simulink model "PassCarModel_RL_config"  (R2024b)
settings: Solver=FixedStepAuto  StartTime=0.0  StopTime=Tf  FixedStep=.001  RelTol=1e-2
StartFcn:
  | %tic
StopFcn:
  | %toc
model workspace (MAT data in the model file):
  AverageTimeInterval = 0.5
  Downshift_Speeds = [9.5625 12.9375 16.3125 19.6875 23.0625 26.4375 29.8125 33.1875 36.5625 39.9375 43.3125 46.6875 ... (28 elements, 4x7)]
  EEC_Counter : Simulink.Parameter (value not decoded)
  EngRevLim = 7000
  FuzzOffset : Simulink.Parameter (value not decoded)
  FuzzRange : Simulink.Parameter (value not decoded)
  Fuzzing : Simulink.Parameter (value not decoded)
  Pedal_Positions = [0.1 0.4 0.5 0.9]
  TrackPoints = [0 36.336 72.672 109.008 145.344 181.68 218.016 254.352 290.688 327.024 363.36 403.196036522 ... (360 elements, 120x3)]
  Upshift_Speeds = [12.9375 16.3125 19.6875 33 26.4375 29.8125 33.1875 52.5 39.9375 43.3125 46.6875 77.25 ... (28 elements, 4x7)]
  VEH : object (value not decoded)
  gradbp : Simulink.Parameter (value not decoded)
  origin : Simulink.Parameter (value not decoded)
  rayDirections = [0 0 0 0 0 0 0 0 0 0 0 0 ... (363 elements, 121x3)]
  rayLengths = [20 20 20 20 20 20 20 20 20 20 20 20 ... (121 elements, 121x1)]
  rayOrigins = [0.5 0.4 0.3 0.2 0.1 0 -0.1 -0.2 -0.3 -0.4 -0.5 0.5 ... (363 elements, 121x3)]
  theta : Simulink.Parameter (value not decoded)
  totalDistance : Simulink.Parameter (value not decoded)
  vel_profile3 : Simulink.Parameter (value not decoded)
  xEast : Simulink.Parameter (value not decoded)
  yNorth : Simulink.Parameter (value not decoded)
symbols that are objects in the model workspace (value not decoded): gradbp, origin, theta, totalDistance, VEH, vel_profile3, xEast, yNorth
undefined symbols (not defined in the file or in its folder): DecelR, DiscIntNeverNeededParam, dspblkCoreblockFVToolHelper, FO_max, FO_min, FR_max, FR_min, gcbh, ODevR, Sim3dSensor, Ts
libraries: simulink x20, dspstat3 x8, autolibutils x6, sim3dgroundtruthsensorlib x2, rllib x1, slpidlib x1, autolibtranscontrolscommon x1, vehdynlibdriver x1, sharedtransform x1, vehdynlibviscommon x1, vehdynlibsens x1
(part 2 of 5)

== system PassCarModel_RL_config/Controllers and CAN network/CAN/BrakeController ==
  Fuzzing : Inport
  VehDataBus : Inport  Port=2
  Bus Creator1 : BusCreator  Inputs=6
  Bus Selector3 : BusSelector  OutputSignals=Cntrl.Brake.ABSFlag,Cntrl.Brake.TCSFlag,Driveline.BrkPrs,Cntrl.Brake.BrkPrsCmd,Wheels.TireFrame.Omega
  EBC1 : Subsystem
  EBC2 : Subsystem
  EBC3 : Subsystem
  EBC4 : Subsystem
  NoiseGenerator : Subsystem
  BrakeController : Outport
  wires:
  VehDataBus/1 -> NoiseGenerator/1(In1), Bus Selector3/1
  Bus Selector3/1 -> EBC1/1(ABSFlagIn)  "<ABSFlag>"
  Bus Selector3/2 -> EBC1/2(TCSFlagIn)  "<TCSFlag>"
  EBC1/1(ABSFlag) -> Bus Creator1/1
  Bus Selector3/3 -> EBC2/1(<BrkPrs>)  "<BrkPrs>"
  EBC2/1(BrkPrs) -> Bus Creator1/3
  Bus Selector3/4 -> EBC3/1(<BrkPrsCmd>)  "<BrkPrsCmd>"
  EBC3/1(BrkPrsCmd) -> Bus Creator1/4
  Bus Selector3/5 -> EBC4/1(<Omega>)  "<Omega>"
  EBC4/1(Omega) -> Bus Creator1/5
  Bus Creator1/1 -> BrakeController/1
  EBC1/2(TCSFlag) -> Bus Creator1/2
  EBC4/2(OmegaFuzz) -> Bus Creator1/6
  NoiseGenerator/1(Out2) -> EBC4/2(Enabled)
  NoiseGenerator/2(Out3) -> EBC4/3(Noise)  "Noise"
  Fuzzing/1 -> NoiseGenerator/2(Fuzzing)

== system PassCarModel_RL_config/Controllers and CAN network/CAN/CentralController ==
  VehDataBus : Inport
  Bus Creator : BusCreator  Inputs=6
  ECC1 : Subsystem
  ECC2 : Subsystem
  CentralController : Outport
  wires:
  VehDataBus/1 -> ECC1/1(In1), ECC2/1(In1)
  Bus Creator/1 -> CentralController/1
  ECC1/1(AccelPedalPos) -> Bus Creator/1
  ECC1/2(BrakePedalPos) -> Bus Creator/2
  ECC1/3(DriveMode) -> Bus Creator/3
  ECC1/4(SteerWheelPos) -> Bus Creator/4
  ECC2/1(PassCarGPSLat) -> Bus Creator/5
  ECC2/2(PassCarGPSLon) -> Bus Creator/6

== system PassCarModel_RL_config/Controllers and CAN network/CAN/EngineController ==
  VehDataBus : Inport
  Bus Creator : BusCreator  Inputs=3
  Bus Selector5 : BusSelector  OutputSignals=Engine.EngTrq,Cntrl.ECU.EngTrqCmd,Driveline.EngSpd
  EngDemandTorque1 : Subsystem
  EngineSpeed1 : Subsystem
  EngineTorque1 : Subsystem
  Signal Specification1 : SignalSpecification  Unit=rpm
  Signal Specification2 : SignalSpecification  Unit=rad/s
  Signal Specification3 : SignalSpecification  Unit=rad/s
  Signal Specification4 : SignalSpecification  Unit=rpm
  Unit Conversion1 : UnitConversion
  Unit Conversion2 : UnitConversion
  EngineController : Outport
  wires:
  Bus Selector5/1 -> EngineTorque1/1(In1)  "<EngTrq>"
  EngDemandTorque1/1(Out2) -> Bus Creator/2  "EngTrqCmd"
  Unit Conversion2/1 -> Signal Specification1/1
  Signal Specification2/1 -> Unit Conversion2/1
  Signal Specification1/1 -> EngineSpeed1/1(In1)
  EngineSpeed1/1(Out2) -> Signal Specification4/1  "EngSpeed"
  Bus Selector5/3 -> Signal Specification2/1  "<EngSpd>"
  EngineTorque1/1(Out2) -> Bus Creator/1  "EngTrq"
  Bus Selector5/2 -> EngDemandTorque1/1(In1)  "<EngTrqCmd>"
  VehDataBus/1 -> Bus Selector5/1
  Bus Creator/1 -> EngineController/1
  Unit Conversion1/1 -> Signal Specification3/1
  Signal Specification3/1 -> Bus Creator/3  "EngSpd"
  Signal Specification4/1 -> Unit Conversion1/1

== system PassCarModel_RL_config/Controllers and CAN network/CAN/TransmissionController ==
  VehDataBus : Inport
  Bus Creator : BusCreator  Inputs=3
  Bus Selector3 : BusSelector  OutputSignals=Driveline.Gear,Driveline.PropShftSpd,Cntrl.Transmission.GearCmd
  Gear2 : Subsystem
  Gear3 : Subsystem
  Signal Specification1 : SignalSpecification  Unit=rad/s
  Signal Specification2 : SignalSpecification  Unit=rpm
  Signal Specification3 : SignalSpecification  Unit=rpm
  TransOutputShaftSpeed1 : Subsystem
  Unit Conversion1 : UnitConversion
  Unit Conversion3 : UnitConversion
  TransmissionController : Outport
  wires:
  Gear2/1(Out2) -> Bus Creator/1  "Gear"
  Unit Conversion3/1 -> Signal Specification3/1
  Bus Selector3/2 -> Unit Conversion3/1  "<PropShftSpd>"
  Bus Selector3/1 -> Gear2/1(In1)  "<Gear>"
  Bus Selector3/3 -> Gear3/1(In1)  "<GearCmd>"
  Gear3/1(Out2) -> Bus Creator/3  "GearCmd"
  Signal Specification3/1 -> TransOutputShaftSpeed1/1(In1)
  VehDataBus/1 -> Bus Selector3/1
  Bus Creator/1 -> TransmissionController/1
  Signal Specification2/1 -> Unit Conversion1/1
  Unit Conversion1/1 -> Signal Specification1/1
  TransOutputShaftSpeed1/1(Out2) -> Signal Specification2/1  "PropShftSpd"
  Signal Specification1/1 -> Bus Creator/2  "PrpShftSpd"

== system PassCarModel_RL_config/Controllers and CAN network/Controllers/ADCMode ==
  In1 : Inport
  Bus Selector3 : BusSelector  OutputSignals=Driver.AccFdbk,Driver.DecelFdbk,Driver.SteerFdbk,Driver.GearFdbk,Wheels.Omega,IMU.Acc,IMU.pqr
  <AccFdbk> : Outport
  <DecelFdbk> : Outport  Port=2
  <SteerFdbk> : Outport  Port=3
  <GearFdbk> : Outport  Port=4
  <Omega> : Outport  Port=5
  <Acc> : Outport  Port=6
  <pqr> : Outport  Port=7
  wires:
  Bus Selector3/2 -> <DecelFdbk>/1  "<DecelFdbk>"
  Bus Selector3/6 -> <Acc>/1  "<Acc>"
  Bus Selector3/7 -> <pqr>/1  "<pqr>"
  In1/1 -> Bus Selector3/1
  Bus Selector3/3 -> <SteerFdbk>/1  "<SteerFdbk>"
  Bus Selector3/4 -> <GearFdbk>/1  "<GearFdbk>"
  Bus Selector3/1 -> <AccFdbk>/1  "<AccFdbk>"
  Bus Selector3/5 -> <Omega>/1  "<Omega>"

== system PassCarModel_RL_config/Controllers and CAN network/Controllers/Active Differential Control ==
  note: 1) Add Subsystem or Model blocks as valid variant choices.
      | 2) You cannot connect blocks at this level. At simulation, connectivity is automatically
      | determined, based on the active variant and port name matching.
  Accel : Inport
  BrkCmd : Inport  Port=2
  Steer : Inport  Port=3
  GearFdbk : Inport  Port=4
  Omega : Inport  Port=5  Unit=rad/s
  axayaz : Inport  Port=6
  pqr : Inport  Port=7
  No Control : Subsystem  VariantControl=0
  Rear Diff Controller : Subsystem  TreatAsAtomicUnit=on  SystemSampleTime=.01  VariantControl=1
  DiffPrsCmd : Outport  VectorParamsAs1DForOutWhenUnconnected=off
  TrqCmd : Outport  Port=2  VectorParamsAs1DForOutWhenUnconnected=off

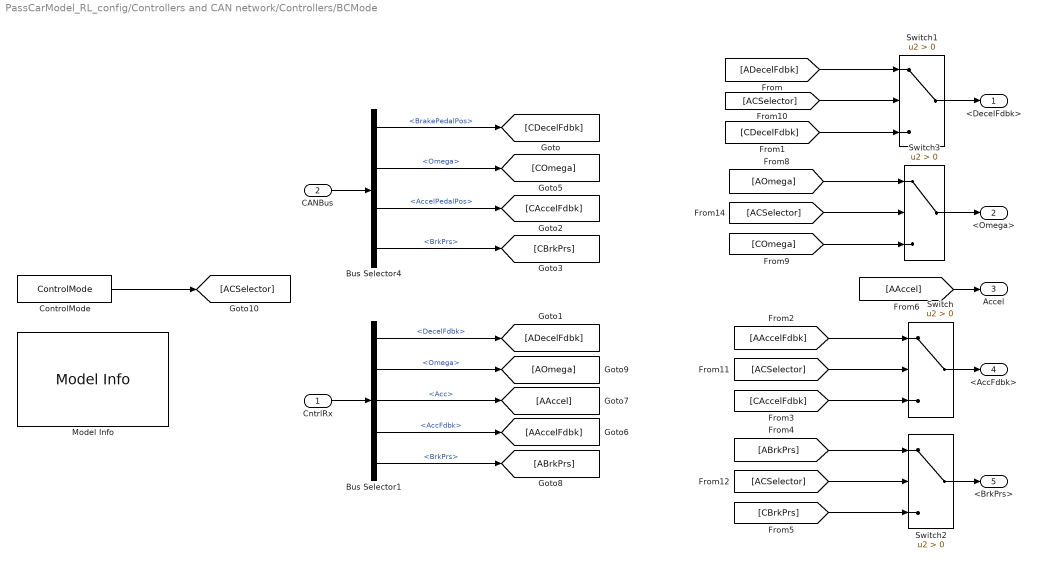
== system PassCarModel_RL_config/Controllers and CAN network/Controllers/BCMode ==
  CntrlRx : Inport
  CANBus : Inport  Port=2
  Bus Selector1 : BusSelector  OutputSignals=Driver.DecelFdbk,Wheels.Omega,IMU.Acc,Driver.AccFdbk,Wheels.BrkPrs
  Bus Selector4 : BusSelector  OutputSignals=CentralController.BrakePedalPos,BrakeController.Omega,CentralController.AccelPedalPos,BrakeController.BrkPrs
  ControlMode : Constant  Value=ControlMode
  Model Info : simulink/Model-Wide Utilities/Model Info  Description=|  Frame=on  DisplayStringWithTags=|  HorizontalTextAlignment=Center  LeftAlignmentValue=0.5
      Description=|
      | CAN == 1
      | Analogue == 0
      DisplayStringWithTags=|
      | CAN == 0
      | Analogue == 1
  Switch{,1..3} (4 alike) : Switch  Criteria=u2 > Threshold  SaturateOnIntegerOverflow=off  InputSameDT=off
  <DecelFdbk> : Outport
  <Omega> : Outport  Port=2
  Accel : Outport  Port=3
  <AccFdbk> : Outport  Port=4
  <BrkPrs> : Outport  Port=5
  wires:
  CANBus/1 -> Bus Selector4/1
  CntrlRx/1 -> Bus Selector1/1
  Bus Selector4/4 -> [CBrkPrs]  "<BrkPrs>"
  Bus Selector4/1 -> [CDecelFdbk]  "<BrakePedalPos>"
  Switch1/1 -> <DecelFdbk>/1
  Bus Selector4/2 -> [COmega]  "<Omega>"
  Bus Selector1/4 -> [AAccelFdbk]  "<AccFdbk>"
  Bus Selector1/1 -> [ADecelFdbk]  "<DecelFdbk>"
  Bus Selector1/2 -> [AOmega]  "<Omega>"
  Switch/1 -> <AccFdbk>/1
  Switch2/1 -> <BrkPrs>/1
  Switch3/1 -> <Omega>/1
  [ADecelFdbk] -> Switch1/1
  [CDecelFdbk] -> Switch1/3
  [AAccelFdbk] -> Switch/1
  [CAccelFdbk] -> Switch/3
  [ABrkPrs] -> Switch2/1
  [CBrkPrs] -> Switch2/3
  [AOmega] -> Switch3/1
  [COmega] -> Switch3/3
  ControlMode/1 -> [ACSelector]
  [ACSelector] -> Switch1/2
  [ACSelector] -> Switch/2
  [ACSelector] -> Switch2/2
  [ACSelector] -> Switch3/2
  Bus Selector1/3 -> [AAccel]  "<Acc>"
  Bus Selector1/5 -> [ABrkPrs]  "<BrkPrs>"
  [AAccel] -> Accel/1
  Bus Selector4/3 -> [CAccelFdbk]  "<AccelPedalPos>"

== system PassCarModel_RL_config/Controllers and CAN network/Controllers/Brake Pressure Control ==
  note: 1) Add Subsystem or Model blocks as valid variant choices.
      | 2) You cannot connect blocks at this level. At simulation, connectivity is automatically
      | determined, based on the active variant and port name matching.
  DecelFdbk : Inport
  Omega : Inport  Port=2
  Accel : Inport  Port=3
  AccelFdbk : Inport  Port=4
  BrkPrs : Inport  Port=5
  Bang Bang ABS : Subsystem  VariantControl=1
  Five-State ABS and TCS : Subsystem  VariantControl=2
  Open Loop : Subsystem  VariantControl=0
  Slip control : Subsystem  VariantControl=Slip control
  ABSFlag : Outport  VectorParamsAs1DForOutWhenUnconnected=off
  BrkPrsCmd : Outport  Port=2  VectorParamsAs1DForOutWhenUnconnected=off
  TCSFlag : Outport  Port=3  VectorParamsAs1DForOutWhenUnconnected=off

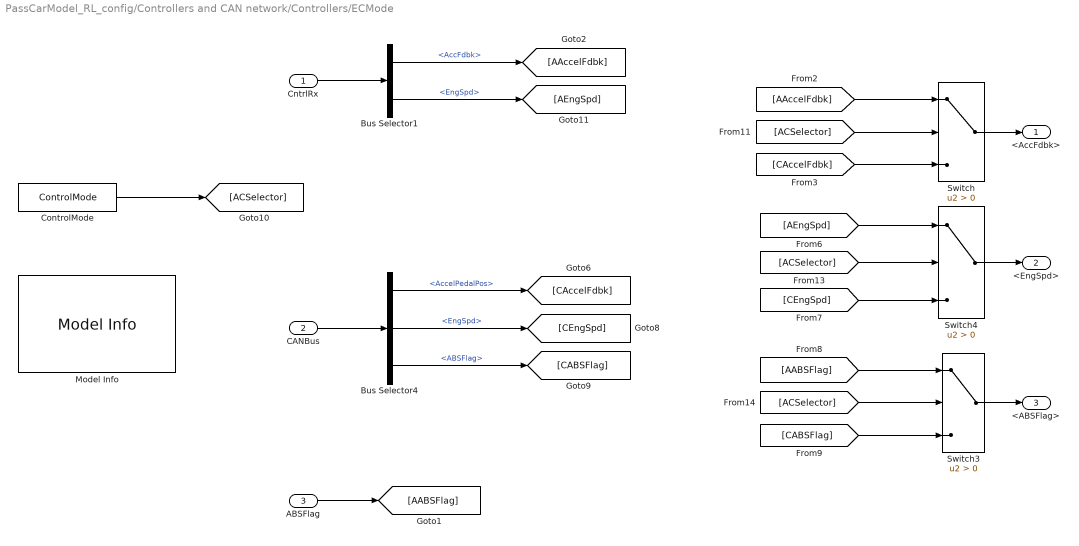
== system PassCarModel_RL_config/Controllers and CAN network/Controllers/ECMode ==
  CntrlRx : Inport
  CANBus : Inport  Port=2
  ABSFlag : Inport  Port=3
  Bus Selector1 : BusSelector  OutputSignals=Driver.AccFdbk,Engine.EngSpd
  Bus Selector4 : BusSelector  OutputSignals=CentralController.AccelPedalPos,EngineController.EngSpd,BrakeController.ABSFlag
  ControlMode : Constant  Value=ControlMode
  Model Info : simulink/Model-Wide Utilities/Model Info  Description=|  Frame=on  DisplayStringWithTags=|  HorizontalTextAlignment=Center  LeftAlignmentValue=0.5
      Description=|
      | CAN == 1
      | Analogue == 0
      DisplayStringWithTags=|
      | CAN == 0
      | Analogue == 1
  Switch : Switch  Criteria=u2 > Threshold  SaturateOnIntegerOverflow=off  InputSameDT=off
  Switch3 : Switch  Criteria=u2 > Threshold  SaturateOnIntegerOverflow=off  InputSameDT=off
  Switch4 : Switch  Criteria=u2 > Threshold  SaturateOnIntegerOverflow=off  InputSameDT=off
  <AccFdbk> : Outport
  <EngSpd> : Outport  Port=2  Unit=rad/s  LockScale=on
  <ABSFlag> : Outport  Port=3
  wires:
  Bus Selector4/3 -> [CABSFlag]  "<ABSFlag>"
  Bus Selector4/2 -> [CEngSpd]  "<EngSpd>"
  Bus Selector4/1 -> [CAccelFdbk]  "<AccelPedalPos>"
  Bus Selector1/2 -> [AEngSpd]  "<EngSpd>"
  Bus Selector1/1 -> [AAccelFdbk]  "<AccFdbk>"
  CANBus/1 -> Bus Selector4/1
  CntrlRx/1 -> Bus Selector1/1
  Switch/1 -> <AccFdbk>/1
  Switch3/1 -> <ABSFlag>/1
  [AAccelFdbk] -> Switch/1
  [CAccelFdbk] -> Switch/3
  [AEngSpd] -> Switch4/1
  [CEngSpd] -> Switch4/3
  [AABSFlag] -> Switch3/1
  [CABSFlag] -> Switch3/3
  ControlMode/1 -> [ACSelector]
  [ACSelector] -> Switch/2
  [ACSelector] -> Switch4/2
  [ACSelector] -> Switch3/2
  ABSFlag/1 -> [AABSFlag]
  Switch4/1 -> <EngSpd>/1

== system PassCarModel_RL_config/Controllers and CAN network/Controllers/ECU ==
  DiffTrqCmd : Inport
  <Accel> : Inport  Port=2
  EngSpd : Inport  Port=3
  ABSFlag : Inport  Port=4
  First Order Hold : FirstOrderHold  ErrorTolerance=100
  Torque Cmd : Subsystem  TreatAsAtomicUnit=on  SystemSampleTime=.01
  EngTrqCmd : Outport  VectorParamsAs1DForOutWhenUnconnected=off
  wires:
  First Order Hold/1 -> EngTrqCmd/1
  DiffTrqCmd/1 -> Torque Cmd/1(DiffTrqCmd)
  <Accel>/1 -> Torque Cmd/2(<Accel>)
  EngSpd/1 -> Torque Cmd/3(EngSpd)
  Torque Cmd/1(EngTrqCmd) -> First Order Hold/1
  ABSFlag/1 -> Torque Cmd/4(ABSFlag)

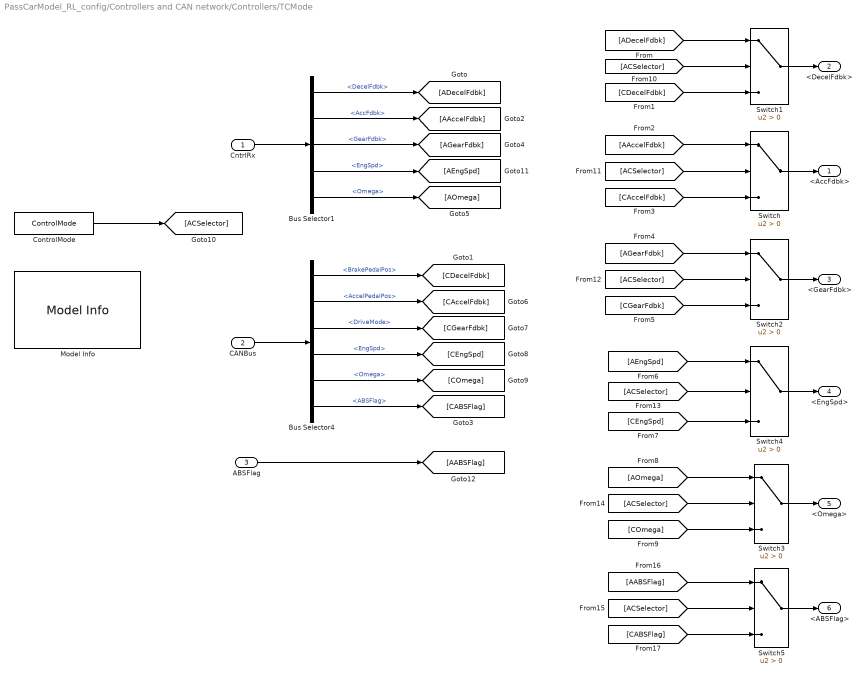
== system PassCarModel_RL_config/Controllers and CAN network/Controllers/TCMode ==
  CntrlRx : Inport
  CANBus : Inport  Port=2
  ABSFlag : Inport  Port=3
  Bus Selector1 : BusSelector  OutputSignals=Driver.DecelFdbk,Driver.AccFdbk,Driver.GearFdbk,Engine.EngSpd,Wheels.Omega
  Bus Selector4 : BusSelector  OutputSignals=CentralController.BrakePedalPos,CentralController.AccelPedalPos,CentralController.DriveMode,EngineController.EngSpd,BrakeController.Omega,BrakeController.ABSFlag
  ControlMode : Constant  Value=ControlMode
  Model Info : simulink/Model-Wide Utilities/Model Info  Description=|  Frame=on  DisplayStringWithTags=|  HorizontalTextAlignment=Center  LeftAlignmentValue=0.5
      Description=|
      | CAN == 1
      | Analogue == 0
      DisplayStringWithTags=|
      | CAN == 0
      | Analogue == 1
  Switch{,1..5} (6 alike) : Switch  Criteria=u2 > Threshold  SaturateOnIntegerOverflow=off  InputSameDT=off
  <AccFdbk> : Outport
  <DecelFdbk> : Outport  Port=2
  <GearFdbk> : Outport  Port=3
  <EngSpd> : Outport  Port=4
  <Omega> : Outport  Port=5
  <ABSFlag> : Outport  Port=6
  wires:
  [ACSelector] -> Switch3/2
  [ACSelector] -> Switch4/2
  [ACSelector] -> Switch2/2
  [ACSelector] -> Switch/2
  [ACSelector] -> Switch1/2
  ControlMode/1 -> [ACSelector]
  [COmega] -> Switch3/3
  [AOmega] -> Switch3/1
  [CEngSpd] -> Switch4/3
  [AEngSpd] -> Switch4/1
  [CGearFdbk] -> Switch2/3
  [AGearFdbk] -> Switch2/1
  [CAccelFdbk] -> Switch/3
  [AAccelFdbk] -> Switch/1
  [CDecelFdbk] -> Switch1/3
  [ADecelFdbk] -> Switch1/1
  Switch3/1 -> <Omega>/1
  Switch2/1 -> <GearFdbk>/1
  Switch/1 -> <AccFdbk>/1
  Switch4/1 -> <EngSpd>/1
  Switch1/1 -> <DecelFdbk>/1
  CntrlRx/1 -> Bus Selector1/1
  CANBus/1 -> Bus Selector4/1
  Bus Selector1/1 -> [ADecelFdbk]  "<DecelFdbk>"
  Bus Selector1/2 -> [AAccelFdbk]  "<AccFdbk>"
  Bus Selector1/3 -> [AGearFdbk]  "<GearFdbk>"
  Bus Selector1/4 -> [AEngSpd]  "<EngSpd>"
  Bus Selector1/5 -> [AOmega]  "<Omega>"
  Bus Selector4/1 -> [CDecelFdbk]  "<BrakePedalPos>"
  Bus Selector4/2 -> [CAccelFdbk]  "<AccelPedalPos>"
  Bus Selector4/3 -> [CGearFdbk]  "<DriveMode>"
  Bus Selector4/4 -> [CEngSpd]  "<EngSpd>"
  Bus Selector4/5 -> [COmega]  "<Omega>"
  Bus Selector4/6 -> [CABSFlag]  "<ABSFlag>"
  Switch5/1 -> <ABSFlag>/1
  [AABSFlag] -> Switch5/1
  [CABSFlag] -> Switch5/3
  [ACSelector] -> Switch5/2
  ABSFlag/1 -> [AABSFlag]

== system PassCarModel_RL_config/Controllers and CAN network/Controllers/Transmission Controller ==
  Accel : Inport
  BrkCmd : Inport  Port=2
  GearReq : Inport  Port=3
  EngSpd : Inport  Port=4
  Omega : Inport  Port=5  Unit=rad/s
  ABSFlag : Inport  Port=6
  UpReq : Inport  Port=7
  DownReq : Inport  Port=8  Unit=rad/s
  Driver - No Clutch : Subsystem  VariantControl=1
  PRNDL Controller : Subsystem  VariantControl=3
  Paddles : Subsystem  VariantControl=2
  Transmission Controller : Subsystem  VariantControl=0
  " Gear" : Outport  VectorParamsAs1DForOutWhenUnconnected=off

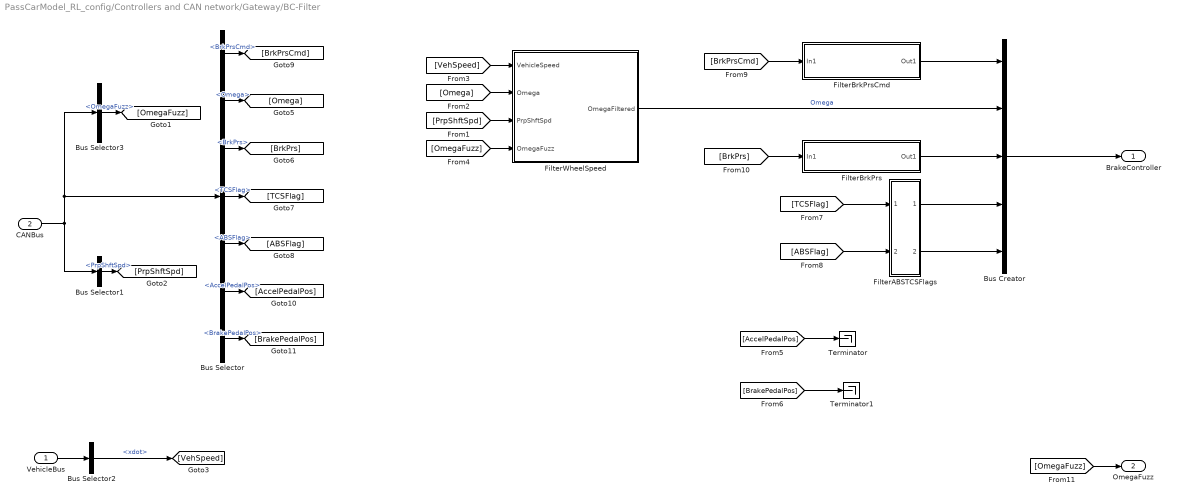
== system PassCarModel_RL_config/Controllers and CAN network/Gateway/BC-Filter ==
  VehicleBus : Inport
  CANBus : Inport  Port=2
  Bus Creator : BusCreator  Inputs=5
  Bus Selector : BusSelector  OutputSignals=BrakeController.BrkPrsCmd,BrakeController.Omega,BrakeController.BrkPrs,BrakeController.TCSFlag,BrakeController.ABSFlag,CentralController.AccelPedalPos,CentralController.BrakePedalPos
  Bus Selector1 : BusSelector  OutputSignals=TransmissionController.PrpShftSpd
  Bus Selector2 : BusSelector  OutputSignals=Body.BdyFrm.Cg.Vel.xdot
  Bus Selector3 : BusSelector  OutputSignals=BrakeController.OmegaFuzz
  FilterABSTCSFlags : Subsystem
  FilterBrkPrs : Subsystem
  FilterBrkPrsCmd : Subsystem
  FilterWheelSpeed : Subsystem
  Terminator : Terminator
  Terminator1 : Terminator
  BrakeController : Outport
  OmegaFuzz : Outport  Port=2
  wires:
  CANBus/1 -> Bus Selector1/1, Bus Selector/1, Bus Selector3/1
  Bus Selector/1 -> [BrkPrsCmd]  "<BrkPrsCmd>"
  Bus Creator/1 -> BrakeController/1
  FilterWheelSpeed/1(OmegaFiltered) -> Bus Creator/2  "Omega"
  FilterBrkPrsCmd/1(Out1) -> Bus Creator/1
  FilterBrkPrs/1(Out1) -> Bus Creator/3
  FilterABSTCSFlags/1(Out1) -> Bus Creator/4
  FilterABSTCSFlags/2(Out2) -> Bus Creator/5
  VehicleBus/1 -> Bus Selector2/1
  [VehSpeed] -> FilterWheelSpeed/1(VehicleSpeed)
  Bus Selector1/1 -> [PrpShftSpd]  "<PrpShftSpd>"
  [PrpShftSpd] -> FilterWheelSpeed/3(PrpShftSpd)
  Bus Selector/6 -> [AccelPedalPos]  "<AccelPedalPos>"
  Bus Selector/7 -> [BrakePedalPos]  "<BrakePedalPos>"
  Bus Selector3/1 -> [OmegaFuzz]  "<OmegaFuzz>"
  Bus Selector/2 -> [Omega]  "<Omega>"
  Bus Selector/3 -> [BrkPrs]  "<BrkPrs>"
  Bus Selector/4 -> [TCSFlag]  "<TCSFlag>"
  Bus Selector/5 -> [ABSFlag]  "<ABSFlag>"
  [Omega] -> FilterWheelSpeed/2(Omega)
  [OmegaFuzz] -> FilterWheelSpeed/4(OmegaFuzz)
  [TCSFlag] -> FilterABSTCSFlags/1(In1)
  [ABSFlag] -> FilterABSTCSFlags/2(In2)
  [BrkPrsCmd] -> FilterBrkPrsCmd/1(In1)
  [BrkPrs] -> FilterBrkPrs/1(In1)
  Bus Selector2/1 -> [VehSpeed]  "<xdot>"
  [AccelPedalPos] -> Terminator/1
  [BrakePedalPos] -> Terminator1/1
  [OmegaFuzz] -> OmegaFuzz/1

== system PassCarModel_RL_config/Vehicle with driver and environment/Driver/Subsystem ==
  In1 : Inport
  Constant : Constant  Value=true  OutDataTypeStr=boolean
  Constant1 : Constant  Value=500*pi/180
  Constant2 : Constant  Value=110
  Constant3 : Constant  Value=0
  Relational Operator : RelationalOperator  OutDataTypeStr=boolean  RndMeth=Simplest  InputSameDT=off
  Switch : Switch  Criteria=u2 > Threshold  SaturateOnIntegerOverflow=off  InputSameDT=off
  Out1 : Outport
  Out2 : Outport  Port=2
  wires:
  In1/1 -> Relational Operator/1
  Constant3/1 -> Switch/3
  Constant2/1 -> Relational Operator/2
  Constant/1 -> Out1/1
  Constant1/1 -> Switch/1
  Relational Operator/1 -> Switch/2
  Switch/1 -> Out2/1

== system PassCarModel_RL_config/Vehicle with driver and environment/Environment/Ground Feedback ==
  Friction : Inport
  VehFdbk : Inport  Port=2
  3D Engine : Subsystem  VariantControl=1
  Constant : Subsystem  VariantControl=0
  Ground : Outport  VectorParamsAs1DForOutWhenUnconnected=off

== system PassCarModel_RL_config/Vehicle with driver and environment/Environment/Road Track Friction ==
  XWhl : Inport
  YWhl : Inport  Port=2
  Cg : Inport  Port=3
  2D Lookup Tbl for Scaling Fctr (Lambda) : Subsystem  TreatAsAtomicUnit=on
      mask init:
      | [~]=vehdynicon('vehdynblk',gcb);
  Bus Selector : BusSelector  OutputSignals=X,Y
  Cnst Lambda : Constant  Value=ones(4,1).*lambda_g
  Constant1 : Constant  Value=SplitLambdaTrck
  Creating Inertial Frm Bpt : Subsystem
  En at t = 0 : Subsystem
  "Lambda (t = 0) " : Memory  InitialCondition=ones(4,1).*lambda_g  InheritSampleTime=on
  Switch : Switch  Criteria=u2 > Threshold  SaturateOnIntegerOverflow=off  InputSameDT=off
  FricCoeffLambda : Outport
  wires:
  YWhl/1 -> 2D Lookup Tbl for Scaling Fctr (Lambda)/2(YWhl)
  XWhl/1 -> 2D Lookup Tbl for Scaling Fctr (Lambda)/1(XWhl)
  2D Lookup Tbl for Scaling Fctr (Lambda)/1(Lambda for each whl) -> Switch/1
  "Lambda (t = 0) "/1 -> FricCoeffLambda/1
  Switch/1 -> "Lambda (t = 0) "/1
  Cnst Lambda/1 -> Switch/3
  Constant1/1 -> Switch/2
  Cg/1 -> Bus Selector/1
  Creating Inertial Frm Bpt/1(XBpt) -> 2D Lookup Tbl for Scaling Fctr (Lambda)/3(XBpt)
  Creating Inertial Frm Bpt/2(YBpt) -> 2D Lookup Tbl for Scaling Fctr (Lambda)/4(YBpt)
  Bus Selector/1 -> Creating Inertial Frm Bpt/1(XCg)  "<X>"
  Bus Selector/2 -> Creating Inertial Frm Bpt/2(YCg)  "<Y>"
  En at t = 0/1(Out1) -> Creating Inertial Frm Bpt/Enable

== system PassCarModel_RL_config/Vehicle with driver and environment/Environment/Wheel Coordinates ==
  FrntAxlLftX : Inport
  FrntAxlRghtX : Inport  Port=2
  RearAxlLftX : Inport  Port=3
  RearAxlRghtX : Inport  Port=4
  FrntAxlLftY : Inport  Port=5
  FrntAxlRghtY : Inport  Port=6
  RearAxlLftY : Inport  Port=7
  RearAxlRghtY : Inport  Port=8
  Matrix Concatenate : Concatenate  NumInputs=4  Mode=Multidimensional array
  Matrix Concatenate1 : Concatenate  NumInputs=4  Mode=Multidimensional array
  XWhl : Outport
  YWhl : Outport  Port=2
  wires:
  RearAxlRghtX/1 -> Matrix Concatenate/4
  Matrix Concatenate/1 -> XWhl/1
  RearAxlRghtY/1 -> Matrix Concatenate1/4
  RearAxlLftX/1 -> Matrix Concatenate/3
  RearAxlLftY/1 -> Matrix Concatenate1/3
  FrntAxlRghtX/1 -> Matrix Concatenate/2
  FrntAxlRghtY/1 -> Matrix Concatenate1/2
  FrntAxlLftY/1 -> Matrix Concatenate1/1
  FrntAxlLftX/1 -> Matrix Concatenate/1
  Matrix Concatenate1/1 -> YWhl/1

== system PassCarModel_RL_config/Vehicle with driver and environment/Passenger Vehicle/Body, Suspension, Wheels ==
  note: 1) Add additional chassis Model reference blocks as valid variant choices for your specific use cases.
      | 2) You cannot connect blocks at this level. At simulation, connectivity is automatically
      | determined, based on the active variant and port name matching.
  WindXYZ : Inport
  Ground : Inport  Port=2  PortDimensions=4
  DCM : Inport  Port=3
  Friction : Inport  Port=4  PortDimensions=4
  WhlAng : Inport  Port=5
  AxlTrq : Inport  Port=6
  BrkPrs : Inport  Port=7
  PassVeh14DOF : ModelReference  DisableCoverage=on  ModelNameDialog=PassVeh14DOF.slx  VariantControl=3  ModelReferenceVersion=9.49
  PassVeh7DOF : ModelReference  ModelNameDialog=PassVeh7DOF  SimulationMode=Normal  VariantControl=1  ModelReferenceVersion=9.3
  Veh : Outport  VectorParamsAs1DForOutWhenUnconnected=off
  Wheels : Outport  Port=2  VectorParamsAs1DForOutWhenUnconnected=off

== system PassCarModel_RL_config/Vehicle with driver and environment/Passenger Vehicle/Chassis Input ==
  Env : Inport
  Driveline : Inport  Port=2
  Bus Selector1 : BusSelector  OutputSignals=Gnd.z.G_FL_z,Gnd.z.G_FR_z,Gnd.z.G_RL_z,Gnd.z.G_RR_z
  Bus Selector2 : BusSelector  OutputSignals=Wind
  Bus Selector3 : BusSelector  OutputSignals=Gnd.mu.mu_FL,Gnd.mu.mu_FR,Gnd.mu.mu_RL,Gnd.mu.mu_RR
  Bus Selector4 : BusSelector  OutputSignals=WhlAng,AxlTrq,BrkPrs
  Bus Selector5 : BusSelector  OutputSignals=Gnd.DCM
  Vector Concatenate : Concatenate  NumInputs=4
  Vector Concatenate1 : Concatenate  NumInputs=4
  Wind : Outport  VectorParamsAs1DForOutWhenUnconnected=off
  Gnd : Outport  Port=2  VectorParamsAs1DForOutWhenUnconnected=off
  DCM : Outport  Port=3  VectorParamsAs1DForOutWhenUnconnected=off
  mu : Outport  Port=4  VectorParamsAs1DForOutWhenUnconnected=off
  WhlAng : Outport  Port=5  VectorParamsAs1DForOutWhenUnconnected=off
  AxlTrq : Outport  Port=6  VectorParamsAs1DForOutWhenUnconnected=off
  BrkPrs : Outport  Port=7  VectorParamsAs1DForOutWhenUnconnected=off
  wires:
  Env/1 -> Bus Selector5/1, Bus Selector3/1, Bus Selector1/1, Bus Selector2/1
  Bus Selector2/1 -> Wind/1  "<Wind>"
  Bus Selector3/1 -> Vector Concatenate/1  "<mu_FL>"
  Bus Selector3/2 -> Vector Concatenate/2  "<mu_FR>"
  Bus Selector3/3 -> Vector Concatenate/3  "<mu_RL>"
  Bus Selector3/4 -> Vector Concatenate/4  "<mu_RR>"
  Vector Concatenate/1 -> mu/1
  Bus Selector1/1 -> Vector Concatenate1/1  "<G_FL_z>"
  Bus Selector1/2 -> Vector Concatenate1/2  "<G_FR_z>"
  Bus Selector1/3 -> Vector Concatenate1/3  "<G_RL_z>"
  Bus Selector1/4 -> Vector Concatenate1/4  "<G_RR_z>"
  Vector Concatenate1/1 -> Gnd/1
  Driveline/1 -> Bus Selector4/1
  Bus Selector4/2 -> AxlTrq/1  "<AxlTrq>"
  Bus Selector4/1 -> WhlAng/1  "<WhlAng>"
  Bus Selector4/3 -> BrkPrs/1  "<BrkPrs>"
  Bus Selector5/1 -> DCM/1  "<DCM>"

== system PassCarModel_RL_config/Vehicle with driver and environment/Passenger Vehicle/Chassis Output ==
  Veh : Inport
  Wheels : Inport  Port=2
  Out Bus Element4 : Outport  PortName=VehFdbk
  Out Bus Element1 : Outport  Port=2  PortName=WheelsFdbk
  wires:
  Veh/1 -> Out Bus Element4/1
  Wheels/1 -> Out Bus Element1/1

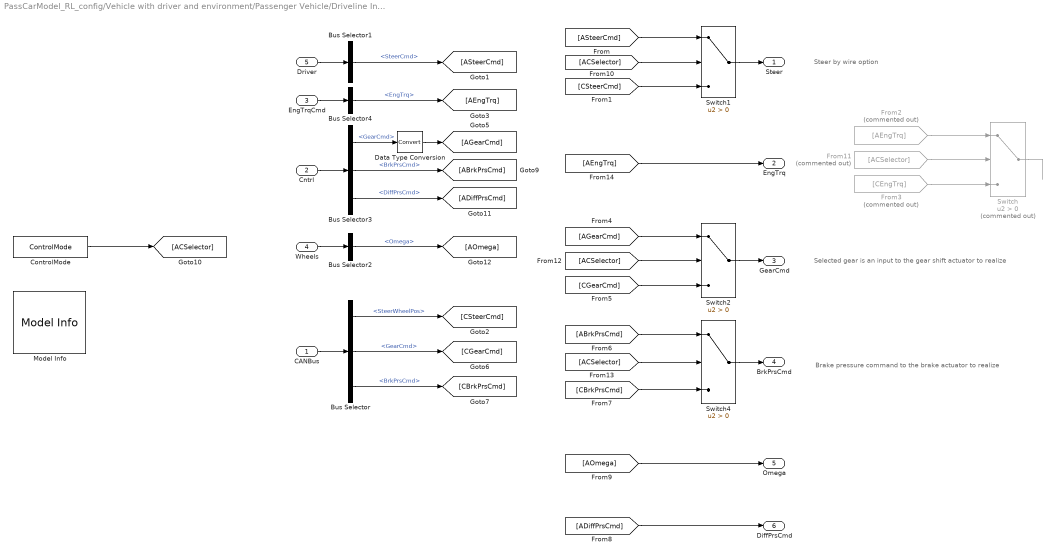
== system PassCarModel_RL_config/Vehicle with driver and environment/Passenger Vehicle/Driveline Input ==
  note: Brake pressure command to the brake actuator to realize
  note: Selected gear is an input to the gear shift actuator to realize
  note: Steer by wire option
  CANBus : Inport
  Cntrl : Inport  Port=2
  EngTrqCmd : Inport  Port=3
  Wheels : Inport  Port=4
  Driver : Inport  Port=5
  Bus Selector : BusSelector  OutputSignals=CentralController.SteerWheelPos,TransmissionController.GearCmd,BrakeController.BrkPrsCmd
  Bus Selector1 : BusSelector  OutputSignals=SteerCmd
  Bus Selector2 : BusSelector  OutputSignals=TireFrame.Omega
  Bus Selector3 : BusSelector  OutputSignals=Transmission.GearCmd,Brake.BrkPrsCmd,Diff.DiffPrsCmd
  Bus Selector4 : BusSelector  OutputSignals=EngTrq
  ControlMode : Constant  Value=ControlMode
  Data Type Conversion : DataTypeConversion  SaturateOnIntegerOverflow=off  RndMeth=Floor
  From11 : From  Commented=on  GotoTag=ACSelector
  From2 : From  Commented=on  GotoTag=AEngTrq
  From3 : From  Commented=on  GotoTag=CEngTrq
  Model Info : simulink/Model-Wide Utilities/Model Info  Frame=on  DisplayStringWithTags=|  HorizontalTextAlignment=Center  LeftAlignmentValue=0.5
      | CAN = 0
      | Analogue = 1
  Switch : Switch  Commented=on  Criteria=u2 > Threshold  SaturateOnIntegerOverflow=off  InputSameDT=off
  Switch1 : Switch  Criteria=u2 > Threshold  SaturateOnIntegerOverflow=off  InputSameDT=off
  Switch2 : Switch  Criteria=u2 > Threshold  SaturateOnIntegerOverflow=off  InputSameDT=off
  Switch4 : Switch  Criteria=u2 > Threshold  SaturateOnIntegerOverflow=off  InputSameDT=off
  Steer : Outport  VectorParamsAs1DForOutWhenUnconnected=off
  EngTrq : Outport  Port=2  VectorParamsAs1DForOutWhenUnconnected=off
  GearCmd : Outport  Port=3  VectorParamsAs1DForOutWhenUnconnected=off
  BrkPrsCmd : Outport  Port=4  VectorParamsAs1DForOutWhenUnconnected=off
  Omega : Outport  Port=5  VectorParamsAs1DForOutWhenUnconnected=off
  DiffPrsCmd : Outport  Port=6  VectorParamsAs1DForOutWhenUnconnected=off
  wires:
  Cntrl/1 -> Bus Selector3/1
  Bus Selector3/1 -> Data Type Conversion/1  "<GearCmd>"
  Driver/1 -> Bus Selector1/1
  Wheels/1 -> Bus Selector2/1
  EngTrqCmd/1 -> Bus Selector4/1
  Bus Selector4/1 -> [AEngTrq]  "<EngTrq>"
  Bus Selector3/3 -> [ADiffPrsCmd]  "<DiffPrsCmd>"
  CANBus/1 -> Bus Selector/1
  ControlMode/1 -> [ACSelector]
  Switch4/1 -> BrkPrsCmd/1
  [CSteerCmd] -> Switch1/3
  [CBrkPrsCmd] -> Switch4/3
  [ACSelector] -> Switch1/2
  [ACSelector] -> Switch4/2
  Switch/1 -> ?
  From11/1 -> Switch/2
  [AGearCmd] -> Switch2/1
  From3/1 -> Switch/3
  [ABrkPrsCmd] -> Switch4/1
  From2/1 -> Switch/1
  Switch2/1 -> GearCmd/1
  [CGearCmd] -> Switch2/3
  Switch1/1 -> Steer/1
  [ASteerCmd] -> Switch1/1
  [ACSelector] -> Switch2/2
  Bus Selector1/1 -> [ASteerCmd]  "<SteerCmd>"
  Bus Selector/1 -> [CSteerCmd]  "<SteerWheelPos>"
  Data Type Conversion/1 -> [AGearCmd]
  Bus Selector/2 -> [CGearCmd]  "<GearCmd>"
  Bus Selector/3 -> [CBrkPrsCmd]  "<BrkPrsCmd>"
  Bus Selector3/2 -> [ABrkPrsCmd]  "<BrkPrsCmd>"
  [ADiffPrsCmd] -> DiffPrsCmd/1
  Bus Selector2/1 -> [AOmega]  "<Omega>"
  [AOmega] -> Omega/1
  [AEngTrq] -> EngTrq/1

== system PassCarModel_RL_config/Vehicle with driver and environment/Passenger Vehicle/Driveline Output ==
  WhlAng : Inport
  AxlTrq : Inport  Port=2
  BrkPrs : Inport  Port=3
  EngSpd : Inport  Port=4
  PropShftSpd : Inport  Port=5
  StrWhlTrq : Inport  Port=6
  Gear : Inport  Port=7
  Bus Creator1 : BusCreator  Inputs=6
  Bus Creator2 : BusCreator  Inputs=1
  Driveline : Outport  VectorParamsAs1DForOutWhenUnconnected=off
  Steering : Outport  Port=2  VectorParamsAs1DForOutWhenUnconnected=off
  wires:
  Bus Creator1/1 -> Driveline/1  "Driveline"
  PropShftSpd/1 -> Bus Creator1/5  "PropShftSpd"
  AxlTrq/1 -> Bus Creator1/2  "AxlTrq"
  WhlAng/1 -> Bus Creator1/1  "WhlAng"
  EngSpd/1 -> Bus Creator1/4  "EngSpd"
  BrkPrs/1 -> Bus Creator1/3  "BrkPrs"
  StrWhlTrq/1 -> Bus Creator2/1  "StrWhlTrq"
  Bus Creator2/1 -> Steering/1  "Steering"
  Gear/1 -> Bus Creator1/6  "Gear"

== system PassCarModel_RL_config/Vehicle with driver and environment/Passenger Vehicle/Engine ==
  note: 1) Add Subsystem or Model blocks as valid variant choices.
      | 2) You cannot connect blocks at this level. At simulation, connectivity is automatically
      | determined, based on the active variant and port name matching.
  TrqCmd : Inport
  EngSpd : Inport  Port=2  Unit=rad/s
  Ideal Mapped Engine : ModelReference  DisableCoverage=on  ModelNameDialog=SiMappedEngineV.slx  VariantControl=0  ModelReferenceVersion=9.26
  EngTrq : Outport  VectorParamsAs1DForOutWhenUnconnected=off

== system PassCarModel_RL_config/Vehicle with driver and environment/Passenger Vehicle/Engine Input ==
  note: CAN = 0
      | Analogue = 1
  note: Engine speed is realized, however it is an input to the model.
      | Engine spped is the output of the transmission, which gets the
      | engine torque as an input, thus engine speed and torque form
      | a physical dynamical system (not control).
  note: Requested torque is received through CAN
  Cntrl : Inport
  Driveline : Inport  Port=2
  CANBus : Inport  Port=3
  Bus Selector : BusSelector  OutputSignals=ECU.EngTrqCmd
  Bus Selector1 : BusSelector  OutputSignals=EngSpd
  Bus Selector2 : BusSelector  OutputSignals=EngineController.EngTrqCmd
  Constant : Constant  Value=ControlMode
  Switch : Switch  Criteria=u2 > Threshold  SaturateOnIntegerOverflow=off  InputSameDT=off
  EngTrqCmd : Outport  VectorParamsAs1DForOutWhenUnconnected=off
  EngSpd : Outport  Port=2  VectorParamsAs1DForOutWhenUnconnected=off
  wires:
  Driveline/1 -> Bus Selector1/1
  Cntrl/1 -> Bus Selector/1
  Constant/1 -> [CMSelector]
  CANBus/1 -> Bus Selector2/1
  Switch/1 -> EngTrqCmd/1
  Bus Selector/1 -> [AEngTrqCmd]  "<EngTrqCmd>"
  Bus Selector1/1 -> EngSpd/1  "<EngSpd>"
  Bus Selector2/1 -> [CEngTrqCmd]  "<EngTrqCmd>"
  [AEngTrqCmd] -> Switch/1
  [CMSelector] -> Switch/2
  [CEngTrqCmd] -> Switch/3

== system PassCarModel_RL_config/Vehicle with driver and environment/Passenger Vehicle/Engine Output ==
  "EngTrq " : Inport
  Bus Creator : BusCreator  Inputs=1
  Eng : Outport  VectorParamsAs1DForOutWhenUnconnected=off
  wires:
  "EngTrq "/1 -> Bus Creator/1  "EngTrq"
  Bus Creator/1 -> Eng/1

== system PassCarModel_RL_config/Vehicle with driver and environment/Passenger Vehicle/Pedal Cluster Input ==
  Driver : Inport
  Driveline : Inport  Port=2
  Steering : Inport  Port=3
  Bus Selector : BusSelector  OutputSignals=SteerCmd,AccelCmd,DecelCmd,GearCmd,GPS
  Bus Selector1 : BusSelector  OutputSignals=BrkPrs
  Bus Selector2 : BusSelector  OutputSignals=StrWhlTrq
  SteerCmd : Outport  VectorParamsAs1DForOutWhenUnconnected=off
  AccelCmd : Outport  Port=2  VectorParamsAs1DForOutWhenUnconnected=off
  DecelCmd : Outport  Port=3  VectorParamsAs1DForOutWhenUnconnected=off
  GearCmd : Outport  Port=4  VectorParamsAs1DForOutWhenUnconnected=off
  BrkPrs : Outport  Port=5  VectorParamsAs1DForOutWhenUnconnected=off
  StrWhlTrq : Outport  Port=6  VectorParamsAs1DForOutWhenUnconnected=off
  GPS : Outport  Port=7  VectorParamsAs1DForOutWhenUnconnected=off
  wires:
  Bus Selector/2 -> AccelCmd/1  "<AccelCmd>"
  Driver/1 -> Bus Selector/1
  Bus Selector/3 -> DecelCmd/1  "<DecelCmd>"
  Bus Selector/4 -> GearCmd/1  "<GearCmd>"
  Bus Selector/1 -> SteerCmd/1  "<SteerCmd>"
  Driveline/1 -> Bus Selector1/1
  Bus Selector1/1 -> BrkPrs/1  "<BrkPrs>"
  Steering/1 -> Bus Selector2/1
  Bus Selector2/1 -> StrWhlTrq/1  "<StrWhlTrq>"
  Bus Selector/5 -> GPS/1  "<GPS>"

== system PassCarModel_RL_config/Vehicle with driver and environment/Passenger Vehicle/Pedal Cluster Output ==
  SteerFdbk : Inport
  AccFdbk : Inport  Port=2
  DecelFdbk : Inport  Port=3
  GearFdbk : Inport  Port=4
  GPSFdbk : Inport  Port=5
  Bus Creator1 : BusCreator  Inputs=5
  Signal Specification : SignalSpecification  Unit=rad
  Signal Specification1 : SignalSpecification  Unit=1
  Signal Specification2 : SignalSpecification  Unit=1
  Signal Specification3 : SignalSpecification  Unit=1
  OperatorFdbk : Outport
  wires:
  Signal Specification1/1 -> Bus Creator1/2  "AccFdbk"
  Signal Specification3/1 -> Bus Creator1/4  "GearFdbk"
  AccFdbk/1 -> Signal Specification1/1
  DecelFdbk/1 -> Signal Specification2/1
  GearFdbk/1 -> Signal Specification3/1
  Signal Specification/1 -> Bus Creator1/1  "SteerFdbk"
  SteerFdbk/1 -> Signal Specification/1
  Bus Creator1/1 -> OperatorFdbk/1
  Signal Specification2/1 -> Bus Creator1/3  "DecelFdbk"
  GPSFdbk/1 -> Bus Creator1/5  "GPSFdbk"

== system PassCarModel_RL_config/Vehicle with driver and environment/Passenger Vehicle/Pedal Cluster and Cabin ==
  note: Placeholder for introducing faults, detailed actuator behavior,
      | interactions of other systems with a human interface such
      | as changes in power steering and braking assistance.
  SteerCmd : Inport
  AccCmd : Inport  Port=2
  DecelCmd : Inport  Port=3
  GearCmd : Inport  Port=4
  BrkPrs : Inport  Port=5
  StrWhlTrq : Inport  Port=6
  GPS : Inport  Port=7
  Brake Pedal : Subsystem
  Dead Zone2 : DeadZone  LowerValue=0  UpperValue=.01  ZeroCross=off
  Dead Zone3 : DeadZone  LowerValue=-.01  UpperValue=.01  ZeroCross=off
  Terminator : Terminator
  Terminator1 : Terminator
  SteerFdbk : Outport
  AccFdbk : Outport  Port=2
  DecelFdbk : Outport  Port=3
  GearFdbk : Outport  Port=4
  GPSFdbk : Outport  Port=5
  wires:
  SteerCmd/1 -> Dead Zone3/1
  AccCmd/1 -> Dead Zone2/1
  DecelCmd/1 -> Brake Pedal/1(DecelCmd)
  GearCmd/1 -> GearFdbk/1
  BrkPrs/1 -> Terminator/1
  StrWhlTrq/1 -> Terminator1/1
  Brake Pedal/1(DecelFdbk) -> DecelFdbk/1
  Dead Zone2/1 -> AccFdbk/1
  Dead Zone3/1 -> SteerFdbk/1
  GPS/1 -> GPSFdbk/1

== system PassCarModel_RL_config/Vehicle with driver and environment/Passenger Vehicle/Steering, Transmission, Driveline and Brakes ==
  note: 1) Add Subsystem or Model blocks as valid variant choices.
      | 2) You cannot connect blocks at this level. At simulation, connectivity is automatically
      | determined, based on the active variant and port name matching.
  SteerHWCmd : Inport
  EngTrq : Inport  Port=2
  GearCmd : Inport  Port=3  OutDataTypeStr=int8
  BrkPrsCmd : Inport  Port=4  PortDimensions=4
  Omega : Inport  Port=5
  DiffPrsCmd : Inport  Port=6
  Driveline Ideal Fixed Gear : ModelReference  DisableCoverage=on  ModelNameDialog=Driveline.slx  VariantControl=0  ModelReferenceVersion=9.23
  WhlAng : Outport  VectorParamsAs1DForOutWhenUnconnected=off
  AxlTrq : Outport  Port=2  VectorParamsAs1DForOutWhenUnconnected=off
  BrkPrs : Outport  Port=3  PortDimensions=4  VectorParamsAs1DForOutWhenUnconnected=off
  EngSpd : Outport  Port=4  Unit=rad/s  VectorParamsAs1DForOutWhenUnconnected=off
  PropShftSpd : Outport  Port=5  VectorParamsAs1DForOutWhenUnconnected=off
  StrWhlTrq : Outport  Port=6  VectorParamsAs1DForOutWhenUnconnected=off
  Gear : Outport  Port=7  VectorParamsAs1DForOutWhenUnconnected=off

== system PassCarModel_RL_config/Controllers and CAN network/CAN/BrakeController/EBC1 ==
  ABSFlagIn : Inport
  TCSFlagIn : Inport  Port=2
  ControlFlag : Subsystem
  ControlFlag1 : Subsystem
  ControlFlag2 : Subsystem
  ControlFlag3 : Subsystem
  ControlFlag4 : Subsystem
  ControlFlag5 : Subsystem
  ControlFlag6 : Subsystem
  ControlFlag7 : Subsystem
  Demux3 : Demux
  Demux4 : Demux
  Mux : Mux
  Mux1 : Mux
  ABSFlag : Outport
  TCSFlag : Outport  Port=2
  wires:
  Demux3/4 -> ControlFlag3/1(In1)
  Demux4/4 -> ControlFlag7/1(In1)
  ControlFlag5/1(Out2) -> Mux1/2
  Demux4/3 -> ControlFlag6/1(In1)
  ControlFlag6/1(Out2) -> Mux1/3
  Demux4/1 -> ControlFlag4/1(In1)
  ControlFlag2/1(Out2) -> Mux/3
  Demux3/1 -> ControlFlag/1(In1)
  ControlFlag1/1(Out2) -> Mux/2
  Mux1/1 -> TCSFlag/1  "TCSFlag"
  Demux3/2 -> ControlFlag1/1(In1)
  ControlFlag3/1(Out2) -> Mux/4
  ControlFlag4/1(Out2) -> Mux1/1
  Demux3/3 -> ControlFlag2/1(In1)
  Mux/1 -> ABSFlag/1  "ABSFlag"
  ControlFlag7/1(Out2) -> Mux1/4
  ControlFlag/1(Out2) -> Mux/1
  Demux4/2 -> ControlFlag5/1(In1)
  ABSFlagIn/1 -> Demux3/1
  TCSFlagIn/1 -> Demux4/1

== system PassCarModel_RL_config/Controllers and CAN network/CAN/BrakeController/EBC2 ==
  <BrkPrs> : Inport
  BrakePressure : Subsystem
  BrakePressure1 : Subsystem
  BrakePressure2 : Subsystem
  BrakePressure3 : Subsystem
  Demux1 : Demux
  Mux2 : Mux
  Signal Specification : SignalSpecification  Unit=kPa
  Signal Specification1 : SignalSpecification  Unit=kPa
  Signal Specification2 : SignalSpecification  Unit=Pa
  Signal Specification5 : SignalSpecification  Unit=Pa
  Unit Conversion : UnitConversion
  Unit Conversion1 : UnitConversion
  BrkPrs : Outport
  wires:
  Demux1/3 -> BrakePressure2/1(In1)
  BrakePressure3/1(Out2) -> Mux2/4
  Signal Specification5/1 -> Unit Conversion/1
  Unit Conversion/1 -> Signal Specification/1
  Demux1/2 -> BrakePressure1/1(In1)
  Signal Specification/1 -> Demux1/1
  Demux1/1 -> BrakePressure/1(In1)
  BrakePressure1/1(Out2) -> Mux2/2
  BrakePressure2/1(Out2) -> Mux2/3
  BrakePressure/1(Out2) -> Mux2/1
  Demux1/4 -> BrakePressure3/1(In1)
  Mux2/1 -> Signal Specification1/1  "BrkPrs"
  <BrkPrs>/1 -> Signal Specification5/1
  Signal Specification1/1 -> Unit Conversion1/1
  Unit Conversion1/1 -> Signal Specification2/1  "BrkPrs"
  Signal Specification2/1 -> BrkPrs/1

== system PassCarModel_RL_config/Controllers and CAN network/CAN/BrakeController/EBC3 ==
  <BrkPrsCmd> : Inport
  BrakePressureCmd : Subsystem
  BrakePressureCmd1 : Subsystem
  BrakePressureCmd2 : Subsystem
  BrakePressureCmd3 : Subsystem
  Demux2 : Demux
  Mux3 : Mux
  BrkPrsCmd : Outport
  wires:
  BrakePressureCmd/1(Out2) -> Mux3/1
  Demux2/2 -> BrakePressureCmd1/1(In1)
  Demux2/1 -> BrakePressureCmd/1(In1)
  BrakePressureCmd1/1(Out2) -> Mux3/2
  Demux2/3 -> BrakePressureCmd2/1(In1)
  BrakePressureCmd2/1(Out2) -> Mux3/3
  BrakePressureCmd3/1(Out2) -> Mux3/4
  Demux2/4 -> BrakePressureCmd3/1(In1)
  Mux3/1 -> BrkPrsCmd/1  "BrkPrsCmd"
  <BrkPrsCmd>/1 -> Demux2/1

== system PassCarModel_RL_config/Controllers and CAN network/CAN/BrakeController/EBC4 ==
  <Omega> : Inport
  Enabled : Inport  Port=2
  Noise : Inport  Port=3
  Demux : Demux
  Gain1 : Gain  Gain=1/(0.29*3.6)
  Gain7 : Gain  Gain=0.29*3.6
  Logical Operator : Logic  Operator=NOT  AllPortsSameDT=off  OutDataTypeStr=boolean
  Mux4 : Mux
  Noise Mixer : Subsystem
  Saturation : Saturate  UpperLimit=400  LowerLimit=0
  Switch : Switch  Criteria=u2 ~= 0  SaturateOnIntegerOverflow=off  InputSameDT=off
  WheelSpeed : Subsystem
  WheelSpeed1 : Subsystem
  WheelSpeed2 : Subsystem
  WheelSpeed3 : Subsystem
  Omega : Outport
  OmegaFuzz : Outport  Port=2
  wires:
  Gain7/1 -> Saturation/1
  WheelSpeed2/1(Out2) -> Mux4/3
  Demux/4 -> WheelSpeed3/1(In1)
  WheelSpeed/1(Out2) -> Mux4/1
  WheelSpeed3/1(Out2) -> Mux4/4
  Demux/2 -> WheelSpeed1/1(In1)
  WheelSpeed1/1(Out2) -> Mux4/2
  Demux/3 -> WheelSpeed2/1(In1)
  Demux/1 -> WheelSpeed/1(In1)
  Mux4/1 -> Switch/1  "Omega"
  <Omega>/1 -> Gain7/1
  Gain1/1 -> Omega/1  "Omega"
  Noise Mixer/1(trigger) -> Logical Operator/1, Switch/2
  Saturation/1 -> Demux/1
  Noise Mixer/2(noise) -> Switch/3
  Noise/1 -> Noise Mixer/2(Noise)
  Enabled/1 -> Noise Mixer/1(Enabled)
  Switch/1 -> Gain1/1  "CAN w noise"
  Logical Operator/1 -> OmegaFuzz/1  "OmegaFuzz"

== system PassCarModel_RL_config/Controllers and CAN network/CAN/BrakeController/NoiseGenerator ==
  In1 : Inport
  Fuzzing : Inport  Port=2
  Bus Selector : BusSelector  OutputSignals=Body.BdyFrm.Cg.Vel.xdot
  Bus Selector1 : BusSelector  OutputSignals=Fuzzing,FuzzingRange,UniformNormal,FuzzingOffset
  Constant1 : Constant  Value=110
  Constant2 : Constant  Value=1100
  Discrete-Time Integrator : DiscreteIntegrator  SampleTime=-1  ICPrevOutput=DiscIntNeverNeededParam  ICPrevScaledInput=DiscIntNeverNeededParam
  Mux : Mux
  Mux1 : Mux
  Product : Product
  Random Number{1..3,8} (4 alike) : RandomNumber
  Relational Operator : RelationalOperator  OutDataTypeStr=boolean  RndMeth=Simplest  InputSameDT=off
  Saturation : Saturate  UpperLimit=inf  LowerLimit=2
  Signal Specification : SignalSpecification  Unit=m
  Sum : Sum  Inputs=|++
  Switch : Switch  Criteria=u2 > Threshold  SaturateOnIntegerOverflow=off  InputSameDT=off
  Switch2 : Switch  Criteria=u2 > Threshold  SaturateOnIntegerOverflow=off  InputSameDT=off
  Uniform Random Number1 : UniformRandomNumber  Minimum=0
  Uniform Random Number2 : UniformRandomNumber  Minimum=0  Seed=1
  Uniform Random Number3 : UniformRandomNumber  Minimum=0  Seed=2
  Uniform Random Number4 : UniformRandomNumber  Minimum=0  Seed=3
  Out2 : Outport
  Out3 : Outport  Port=2
  wires:
  Uniform Random Number3/1 -> Mux/3
  Uniform Random Number2/1 -> Mux/2
  Uniform Random Number1/1 -> Mux/1
  Uniform Random Number4/1 -> Mux/4
  Mux/1 -> Switch2/1
  Bus Selector/1 -> Discrete-Time Integrator/1  "<xdot>"
  Relational Operator/1 -> Out2/1
  In1/1 -> Bus Selector/1
  Signal Specification/1 -> Relational Operator/1
  Discrete-Time Integrator/1 -> Signal Specification/1
  Switch/1 -> Saturation/1
  Product/1 -> Sum/1
  Saturation/1 -> Relational Operator/2
  Bus Selector1/4 -> Sum/2  "<FuzzingOffset>"
  Constant1/1 -> Switch/1
  Constant2/1 -> Switch/3
  Bus Selector1/1 -> Switch/2  "<Fuzzing>"
  Sum/1 -> Out3/1
  Bus Selector1/3 -> Switch2/2  "<UniformNormal>"
  Bus Selector1/2 -> Product/1  "<FuzzingRange>"
  Fuzzing/1 -> Bus Selector1/1
  Switch2/1 -> Product/2
  Random Number2/1 -> Mux1/2
  Random Number1/1 -> Mux1/1
  Random Number8/1 -> Mux1/4
  Random Number3/1 -> Mux1/3
  Mux1/1 -> Switch2/3

== system PassCarModel_RL_config/Controllers and CAN network/CAN/CentralController/ECC1 ==
  In1 : Inport
  Bus Selector7 : BusSelector  OutputSignals=Driver.AccFdbk,Driver.DecelFdbk,Driver.GearFdbk,Driver.SteerFdbk
  ControlSignal2 : Subsystem
  ControlSignal3 : Subsystem
  Gear1 : Subsystem
  Signal Specification1 : SignalSpecification  Unit=rad
  Signal Specification3 : SignalSpecification  Unit=deg
  Signal Specification4 : SignalSpecification  Unit=deg
  SteeringWheelPos1 : Subsystem
  Unit Conversion1 : UnitConversion
  Unit Conversion4 : UnitConversion
  AccelPedalPos : Outport
  BrakePedalPos : Outport  Port=2
  DriveMode : Outport  Port=3
  SteerWheelPos : Outport  Port=4
  wires:
  Bus Selector7/4 -> Unit Conversion4/1  "<SteerFdbk>"
  Unit Conversion4/1 -> Signal Specification4/1
  Bus Selector7/3 -> Gear1/1(In1)  "<GearFdbk>"
  Bus Selector7/1 -> ControlSignal2/1(In1)  "<AccFdbk>"
  Signal Specification4/1 -> SteeringWheelPos1/1(In1)
  Gear1/1(Out2) -> DriveMode/1  "DriveMode"
  Bus Selector7/2 -> ControlSignal3/1(In1)  "<DecelFdbk>"
  In1/1 -> Bus Selector7/1
  ControlSignal2/1(Out2) -> AccelPedalPos/1  "AccelPedalPos"
  SteeringWheelPos1/1(Out2) -> Signal Specification3/1
  ControlSignal3/1(Out2) -> BrakePedalPos/1  "BrakePedalPos"
  Signal Specification3/1 -> Unit Conversion1/1
  Signal Specification1/1 -> SteerWheelPos/1  "SteerWheelPos"
  Unit Conversion1/1 -> Signal Specification1/1

== system PassCarModel_RL_config/Controllers and CAN network/CAN/CentralController/ECC2 ==
  In1 : Inport
  Bus Selector6 : BusSelector  OutputSignals=Driver.GPSFdbk
  Demux5 : Demux  Outputs=2
  GPS coord : Subsystem
  GPS coord1 : Subsystem
  PassCarGPSLat : Outport
  PassCarGPSLon : Outport  Port=2
  wires:
  Bus Selector6/1 -> Demux5/1  "<GPSFdbk>"
  GPS coord1/1("1 ") -> PassCarGPSLon/1  "PassCarGpsLon"
  Demux5/2 -> GPS coord1/1(In1)
  Demux5/1 -> GPS coord/1(In1)
  In1/1 -> Bus Selector6/1
  GPS coord/1(Out2) -> PassCarGPSLat/1  "PassCarGPSLat"

== system PassCarModel_RL_config/Controllers and CAN network/CAN/EngineController/EngDemandTorque1 ==
  note: 16 bit unsigned
      | factor - 0.0078125
      | offset - -100
      | min - -100
      | max - 411.9921875
      | unit - N/A
  In1 : Inport
  Memory : Memory
  Zero-Order Hold : ZeroOrderHold  SampleTime=0.005
  fix point : DataTypeConversion  OutMin=-100  OutMax=411.9921875  OutDataTypeStr=fixdt(0,16,2^(-7),-100)  SaturateOnIntegerOverflow=off  RndMeth=Floor
  Out2 : Outport
  wires:
  In1/1 -> Zero-Order Hold/1
  Memory/1 -> Out2/1
  fix point/1 -> Memory/1
  Zero-Order Hold/1 -> fix point/1

== system PassCarModel_RL_config/Controllers and CAN network/CAN/EngineController/EngineSpeed1 ==
  note: 16 bit unsigned
      | factor - 0.2
      | offset - 0
      | min - 0
      | max - 13107
      | unit - rpm
  In1 : Inport
  Memory : Memory
  Zero-Order Hold : ZeroOrderHold  SampleTime=0.005
  fix point : DataTypeConversion  OutMin=0  OutMax=13107  OutDataTypeStr=fixdt(0,16,0.2,0)  SaturateOnIntegerOverflow=off  RndMeth=Floor
  Out2 : Outport
  wires:
  In1/1 -> Zero-Order Hold/1
  Memory/1 -> Out2/1
  fix point/1 -> Memory/1
  Zero-Order Hold/1 -> fix point/1

== system PassCarModel_RL_config/Controllers and CAN network/CAN/EngineController/EngineTorque1 ==
  note: 16 bit unsigned
      | factor - 0.0078125
      | offset - -200
      | min - -200
      | max - 311.9921875
      | unit - %
  In1 : Inport
  Memory : Memory
  Zero-Order Hold : ZeroOrderHold  SampleTime=0.005
  fix point : DataTypeConversion  OutMin=-200  OutMax=311.9921875  OutDataTypeStr=fixdt(0,16,2^(-7),-200)  SaturateOnIntegerOverflow=off  RndMeth=Floor
  Out2 : Outport
  wires:
  In1/1 -> Zero-Order Hold/1
  Memory/1 -> Out2/1
  fix point/1 -> Memory/1
  Zero-Order Hold/1 -> fix point/1

== system PassCarModel_RL_config/Controllers and CAN network/CAN/TransmissionController/Gear2 ==
  note: 8 bit unsigned
      | factor - 1
      | offset - 0
      | min - -125
      | max - 125
      | unit - deg
  In1 : Inport
  Memory : Memory
  Zero-Order Hold : ZeroOrderHold  SampleTime=0.005
  fix point : DataTypeConversion  OutMin=-125  OutMax=125  OutDataTypeStr=fixdt(0,8,1,-125)  SaturateOnIntegerOverflow=off  RndMeth=Floor
  Out2 : Outport
  wires:
  Zero-Order Hold/1 -> fix point/1
  fix point/1 -> Memory/1
  Memory/1 -> Out2/1
  In1/1 -> Zero-Order Hold/1

== system PassCarModel_RL_config/Controllers and CAN network/CAN/TransmissionController/Gear3 ==
  note: 8 bit unsigned
      | factor - 1
      | offset - 0
      | min - -125
      | max - 125
      | unit - deg
  In1 : Inport
  Memory : Memory
  Zero-Order Hold : ZeroOrderHold  SampleTime=0.005
  fix point : DataTypeConversion  OutMin=-125  OutMax=125  OutDataTypeStr=fixdt(0,8,1,-125)  SaturateOnIntegerOverflow=off  RndMeth=Floor
  Out2 : Outport
  wires:
  Zero-Order Hold/1 -> fix point/1
  fix point/1 -> Memory/1
  Memory/1 -> Out2/1
  In1/1 -> Zero-Order Hold/1

== system PassCarModel_RL_config/Controllers and CAN network/CAN/TransmissionController/TransOutputShaftSpeed1 ==
  note: 16 bit unsigned
      | factor - 0.125
      | offset - 0
      | min - 0
      | max - 8191.875
      | unit - rpm
  In1 : Inport
  Memory : Memory
  Zero-Order Hold : ZeroOrderHold  SampleTime=0.005
  fix point : DataTypeConversion  OutMin=0  OutMax=8191.875  OutDataTypeStr=fixdt(0,16,0.125,0)  SaturateOnIntegerOverflow=off  RndMeth=Floor
  Out2 : Outport
  wires:
  Zero-Order Hold/1 -> fix point/1
  fix point/1 -> Memory/1
  Memory/1 -> Out2/1
  In1/1 -> Zero-Order Hold/1

== system PassCarModel_RL_config/Controllers and CAN network/Controllers/Active Differential Control/No Control ==
  axayaz : Inport
  Steer : Inport  Port=2
  Constant : Constant  Value=0
  Constant1 : Constant  Value=0
  Terminator : Terminator
  Terminator1 : Terminator
  Vector Concatenate2 : Concatenate  NumInputs=4
  DiffPrsCmd : Outport  VectorParamsAs1DForOutWhenUnconnected=off
  TrqCmd : Outport  Port=2  VectorParamsAs1DForOutWhenUnconnected=off
  wires:
  Constant/1 -> Vector Concatenate2/1, Vector Concatenate2/4, Vector Concatenate2/3, Vector Concatenate2/2
  Steer/1 -> Terminator1/1
  Vector Concatenate2/1 -> DiffPrsCmd/1  "DiffPrsCmd"
  axayaz/1 -> Terminator/1
  Constant1/1 -> TrqCmd/1  "TrqCmd"
